simulink model "ADIA"  (R2018b)
settings: Solver=FixedStepDiscrete  StartTime=0.0  StopTime=10.0  FixedStep=0.02  RelTol=1e-3
undefined symbols (not defined in the file or in its folder): ACC_State_Active, ACC_State_BrakeOnly, ACC_State_Suspended, ACC_State_WaitingRise, ADAS_AEBBrakingProg, ADAS_DeclControlReq, ADAS_DriveOff, ADAS_ESCHoldReq_NotHold, ADASDecType_ACC, ADASDecType_AEB, ADIA_ACC_Acceleration_OOR_DecCount_C, ADIA_ACC_Acceleration_OOR_Duration_C, ADIA_ACC_Acceleration_OOR_IncCount_C, ADIA_ACC_Acceleration_OOR_LLim_C, ADIA_ACC_Acceleration_OOR_ULim_C, ADIA_ACC_AccelTrqReq_MixedDia_ULim_C, ADIA_ACC_AccelTrqReq_ULim_C, ADIA_ACC_Deceleration_Mixed_ULim_C, ADIA_ACC_Deceleration_OOR_DecCount_C, ADIA_ACC_Deceleration_OOR_Duration_C, ADIA_ACC_Deceleration_OOR_IncCount_C, ADIA_ACC_Deceleration_OOR_LLim_C, ADIA_ACC_Deceleration_OOR_ULim_C, ADIA_ACC_DriveOff_Distance_C, ADIA_ACC_DriveOff_TimeLim_C, ADIA_ACC_ReqMixed_DecCount_C, ADIA_ACC_ReqMixed_Duration_C, ADIA_ACC_ReqMixed_IncCount_C, ADIA_AccPedalRaw_MaxLim_C, ADIA_AccPedalRaw_MinLim_C, ADIA_ADAS_HoldDecReq_Set_C, ADIA_ADAS_HoldRConfirm_TimeLim_C, ADIA_ADAS_HoldVehSpd_Lim_C, ADIA_AEB_VehSpdDec_LLim_C, ADIA_AEB_VehSpdDec_ULim_C, ADIA_ASWFault_OvrdEn_C, ADIA_ASWFault_OvrdValue_C, ADIA_BatteryOutOfRange_DecCount_C, ADIA_BatteryOutOfRange_Duration_C, ADIA_BatteryOutOfRange_IncCount_C, ADIA_BattVolt_MaxLim_C, ADIA_BattVolt_MinLim_C, ADIA_BCM3_33C_InvBrkLight_DecCount_C, ADIA_BCM3_33C_InvBrkLight_Duration_C, ADIA_BCM3_33C_InvBrkLight_IncCount_C, ADIA_BCM_BattVolt_OvrdEn_C, ADIA_BCM_BattVolt_OvrdVal_C, ADIA_BCM_BrakeLampStaus_OvrdEn_C, ADIA_BCM_BrakeLampStaus_OvrdVal_C, ADIA_BCM_CHMSLStaus_OvrdEn_C, ADIA_BCM_CHMSLStaus_OvrdVal_C, ADIA_BCM_LeftTurnSwSt_OvrdEn_C, ADIA_BCM_LeftTurnSwSt_OvrdVal_C, ADIA_BCM_RightTurnSwSt_OvrdEn_C, ADIA_BCM_RightTurnSwSt_OvrdVal_C, ADIA_BCM_TurnSwFailure_DecCount_C, ADIA_BCM_TurnSwFailure_Duration_C, ADIA_BCM_TurnSwFailure_IncCount_C, ADIA_BSWFault_Ignore_C, ADIA_BSWFault_OvrdEn_C ... (+281)
libraries: simulink x208
(part 6 of 10)

== system ADIA/ADAS_Diagnostics/Diagnostics_Processing/Rationality_Diagnostics/ESC6_123_InvVehDriDirec ==
  Compare To Constant27 : simulink/Logic and Bit Operations/Compare To Constant  relop===  const=3  OutDataTypeStr=boolean
  Constant18 : Constant  Value=Constant_0
  Constant19 : Constant  Value=ADIA_ESC6_123_InvVehDriDirec_DecCount_C
  Constant20 : Constant  Value=ADIA_ESC6_123_InvVehDriDirec_IncCount_C
  Constant21 : Constant  Value=ADIA_ESC6_123_InvVehDriDirec_Duration_C
  Constant22 : Constant  Value=SYS_False
  Counter&Latch : Subsystem
  Data Store Read67 : DataStoreRead  DataStoreName=ADIAve_y_ESC_VehDrivingDirection
  Logical Operator20 : Logic  Operator=NOT  AllPortsSameDT=off  OutDataTypeStr=boolean
  ADIA_DTC_ESC6_123_InvVehDriDirec : Outport
  wires:
  Compare To Constant27/1 -> Logical Operator20/1, Counter&Latch/1(incrcondition)  "Event_OutRangePowStrSta_SetEventStatus19"
  Data Store Read67/1 -> Compare To Constant27/1  "ob_ADIAve_y_ESC_VehDrivingDirection"
  Logical Operator20/1 -> Counter&Latch/3(decrcondition)
  Constant19/1 -> Counter&Latch/4(decvalue)
  Constant20/1 -> Counter&Latch/2(incrvalue)
  Constant18/1 -> Counter&Latch/7(LatchResetCounterVal)
  Constant21/1 -> Counter&Latch/5(maxlimit)
  Constant22/1 -> Counter&Latch/6(reset)
  Counter&Latch/1(Out1) -> ADIA_DTC_ESC6_123_InvVehDriDirec/1

== system ADIA/ADAS_Diagnostics/Diagnostics_Processing/Rationality_Diagnostics/ESC6_123_InvVehHoldStas ==
  Compare To Constant45 : simulink/Logic and Bit Operations/Compare To Constant  relop===  const=3  OutDataTypeStr=boolean
  Constant18 : Constant  Value=Constant_0
  Constant19 : Constant  Value=ADIA_ESC6_123_InvVehHoldStas_DecCount_C
  Constant20 : Constant  Value=ADIA_ESC6_123_InvVehHoldStas_IncCount_C
  Constant21 : Constant  Value=ADIA_ESC6_123_InvVehHoldStas_Duration_C
  Constant22 : Constant  Value=SYS_False
  Counter&Latch : Subsystem
  Data Store Read33 : DataStoreRead  DataStoreName=ADIAve_y_ESC_VehHoldState
  Logical Operator20 : Logic  Operator=NOT  AllPortsSameDT=off  OutDataTypeStr=boolean
  ADIA_DTC_ESC6_123_InvVehHoldStas : Outport
  wires:
  Compare To Constant45/1 -> Counter&Latch/1(incrcondition), Logical Operator20/1  "Event_OutRangeHoldSta_SetEventStatus22"
  Data Store Read33/1 -> Compare To Constant45/1
  Logical Operator20/1 -> Counter&Latch/3(decrcondition)
  Constant19/1 -> Counter&Latch/4(decvalue)
  Constant20/1 -> Counter&Latch/2(incrvalue)
  Constant18/1 -> Counter&Latch/7(LatchResetCounterVal)
  Constant21/1 -> Counter&Latch/5(maxlimit)
  Constant22/1 -> Counter&Latch/6(reset)
  Counter&Latch/1(Out1) -> ADIA_DTC_ESC6_123_InvVehHoldStas/1

== system ADIA/ADAS_Diagnostics/Diagnostics_Processing/Rationality_Diagnostics/Event_Fault_ABSorESC ==
  Compare To Constant8 : simulink/Logic and Bit Operations/Compare To Constant  relop===  const=1  OutDataTypeStr=boolean
  Compare To Constant9 : simulink/Logic and Bit Operations/Compare To Constant  relop===  const=1  OutDataTypeStr=boolean
  Data Store Read52 : DataStoreRead  DataStoreName=ADIAve_y_ESC_ABSValidity
  Data Store Read53 : DataStoreRead  DataStoreName=ADIAve_y_ESC_ESCValidity
  Logical Operator20 : Logic  Operator=OR  AllPortsSameDT=off  OutDataTypeStr=boolean
  "Event_Fault_ABSorESC " : Outport
  wires:
  Data Store Read52/1 -> Compare To Constant8/1
  Compare To Constant9/1 -> Logical Operator20/2  "Event_FaulESCLamp6"
  Data Store Read53/1 -> Compare To Constant9/1
  Logical Operator20/1 -> "Event_Fault_ABSorESC "/1
  Compare To Constant8/1 -> Logical Operator20/1  "Event_FaulABSLamp5"

== system ADIA/ADAS_Diagnostics/Diagnostics_Processing/Rationality_Diagnostics/FRadar_FaultState ==
  Constant18 : Constant  Value=Constant_0
  Constant19 : Constant  Value=ADIA_FRadar_FaultState_DecCount_C
  Constant20 : Constant  Value=ADIA_FRadar_FaultState_IncCount_C
  Constant21 : Constant  Value=ADIA_FRadar_FaultState_Duration_C
  Constant22 : Constant  Value=SYS_False
  Constant37 : Constant  Value=FRadar_State_Sensoring
  Counter&Latch : Subsystem
  Data Store Read74 : DataStoreRead  DataStoreName=ADIAve_y_Radar_State
  Logical Operator20 : Logic  Operator=NOT  AllPortsSameDT=off  OutDataTypeStr=boolean
  Relational Operator37 : RelationalOperator  Operator=~=  OutDataTypeStr=boolean  RndMeth=Simplest
  ADIA_Inner_FRadar_FaultState : Outport
  wires:
  Constant37/1 -> Relational Operator37/2
  Data Store Read74/1 -> Relational Operator37/1  "ob_ADIAve_y_Radar_State"
  Logical Operator20/1 -> Counter&Latch/3(decrcondition)
  Relational Operator37/1 -> Logical Operator20/1, Counter&Latch/1(incrcondition)
  Constant19/1 -> Counter&Latch/4(decvalue)
  Constant20/1 -> Counter&Latch/2(incrvalue)
  Constant18/1 -> Counter&Latch/7(LatchResetCounterVal)
  Constant21/1 -> Counter&Latch/5(maxlimit)
  Constant22/1 -> Counter&Latch/6(reset)
  Counter&Latch/1(Out1) -> ADIA_Inner_FRadar_FaultState/1

== system ADIA/ADAS_Diagnostics/Diagnostics_Processing/Rationality_Diagnostics/MP5_366_OorAEBButton ==
  Compare To Constant50 : simulink/Logic and Bit Operations/Compare To Constant  relop===  const=3  OutDataTypeStr=boolean
  Constant18 : Constant  Value=Constant_0
  Constant19 : Constant  Value=ADIA_MP5_366_OorAEBButton_DecCount_C
  Constant20 : Constant  Value=ADIA_MP5_366_OorAEBButton_IncCount_C
  Constant21 : Constant  Value=ADIA_MP5_366_OorAEBButton_Duration_C
  Constant22 : Constant  Value=SYS_False
  Counter&Latch : Subsystem
  Data Store Read38 : DataStoreRead  DataStoreName=ADIAve_y_MP5_AEBSwitch
  Logical Operator20 : Logic  Operator=NOT  AllPortsSameDT=off  OutDataTypeStr=boolean
  ADIA_DTC_MP5_366_OorAEBButton : Outport
  wires:
  Data Store Read38/1 -> Compare To Constant50/1
  Logical Operator20/1 -> Counter&Latch/3(decrcondition)
  Compare To Constant50/1 -> Logical Operator20/1, Counter&Latch/1(incrcondition)
  Constant19/1 -> Counter&Latch/4(decvalue)
  Constant20/1 -> Counter&Latch/2(incrvalue)
  Constant18/1 -> Counter&Latch/7(LatchResetCounterVal)
  Constant21/1 -> Counter&Latch/5(maxlimit)
  Constant22/1 -> Counter&Latch/6(reset)
  Counter&Latch/1(Out1) -> ADIA_DTC_MP5_366_OorAEBButton/1

== system ADIA/ADAS_Diagnostics/Diagnostics_Processing/Rationality_Diagnostics/MP5_366_OorFCWButton ==
  Compare To Constant51 : simulink/Logic and Bit Operations/Compare To Constant  relop===  const=3  OutDataTypeStr=boolean
  Constant18 : Constant  Value=Constant_0
  Constant19 : Constant  Value=ADIA_MP5_366_OorFCWButton_DecCount_C
  Constant20 : Constant  Value=ADIA_MP5_366_OorFCWButton_IncCount_C
  Constant21 : Constant  Value=ADIA_MP5_366_OorFCWButton_Duration_C
  Constant22 : Constant  Value=SYS_False
  Counter&Latch : Subsystem
  Data Store Read37 : DataStoreRead  DataStoreName=ADIAve_y_MP5_FCWSwitch
  Logical Operator20 : Logic  Operator=NOT  AllPortsSameDT=off  OutDataTypeStr=boolean
  ADIA_DTC_MP5_366_OorFCWButton : Outport
  wires:
  Data Store Read37/1 -> Compare To Constant51/1
  Logical Operator20/1 -> Counter&Latch/3(decrcondition)
  Compare To Constant51/1 -> Counter&Latch/1(incrcondition), Logical Operator20/1
  Constant19/1 -> Counter&Latch/4(decvalue)
  Constant20/1 -> Counter&Latch/2(incrvalue)
  Constant18/1 -> Counter&Latch/7(LatchResetCounterVal)
  Constant21/1 -> Counter&Latch/5(maxlimit)
  Constant22/1 -> Counter&Latch/6(reset)
  Counter&Latch/1(Out1) -> ADIA_DTC_MP5_366_OorFCWButton/1

== system ADIA/ADAS_Diagnostics/Diagnostics_Processing/Rationality_Diagnostics/MP5_413_OorISAMode ==
  Compare To Constant31 : simulink/Logic and Bit Operations/Compare To Constant  relop===  const=3  OutDataTypeStr=boolean
  Constant18 : Constant  Value=Constant_0
  Constant19 : Constant  Value=ADIA_MP5_413_OorISAMode_DecCount_C
  Constant20 : Constant  Value=ADIA_MP5_413_OorISAMode_IncCount_C
  Constant21 : Constant  Value=ADIA_MP5_413_OorISAMode_Duration_C
  Constant22 : Constant  Value=SYS_False
  Counter&Latch : Subsystem
  Data Store Read71 : DataStoreRead  DataStoreName=ADIAve_y_Mp5_ISAMode
  Logical Operator20 : Logic  Operator=NOT  AllPortsSameDT=off  OutDataTypeStr=boolean
  ADIA_DTC_GW_MP5_413_OorISAMode : Outport
  wires:
  Compare To Constant31/1 -> Logical Operator20/1, Counter&Latch/1(incrcondition)  "Event_OutRangePowStrSta_SetEventStatus19"
  Data Store Read71/1 -> Compare To Constant31/1  "ob_ADIAve_y_Mp5_ISAMode"
  Logical Operator20/1 -> Counter&Latch/3(decrcondition)
  Constant19/1 -> Counter&Latch/4(decvalue)
  Constant20/1 -> Counter&Latch/2(incrvalue)
  Constant18/1 -> Counter&Latch/7(LatchResetCounterVal)
  Constant21/1 -> Counter&Latch/5(maxlimit)
  Constant22/1 -> Counter&Latch/6(reset)
  Counter&Latch/1(Out1) -> ADIA_DTC_GW_MP5_413_OorISAMode/1

== system ADIA/ADAS_Diagnostics/Diagnostics_Processing/Rationality_Diagnostics/MP5_413_OorLKAMode ==
  Compare To Constant49 : simulink/Logic and Bit Operations/Compare To Constant  relop=>=  const=6  OutDataTypeStr=boolean
  Constant18 : Constant  Value=Constant_0
  Constant19 : Constant  Value=ADIA_MP5_413_OorLKAMode_DecCount_C
  Constant20 : Constant  Value=ADIA_MP5_413_OorLKAMode_IncCount_C
  Constant21 : Constant  Value=ADIA_MP5_413_OorLKAMode_Duration_C
  Constant22 : Constant  Value=SYS_False
  Counter&Latch : Subsystem
  Data Store Read39 : DataStoreRead  DataStoreName=ADIAve_y_Mp5_LSSMode
  Logical Operator20 : Logic  Operator=NOT  AllPortsSameDT=off  OutDataTypeStr=boolean
  ADIA_DTC_GW_MP5_413_OorLKAMode : Outport
  wires:
  Data Store Read39/1 -> Compare To Constant49/1
  Logical Operator20/1 -> Counter&Latch/3(decrcondition)
  Compare To Constant49/1 -> Counter&Latch/1(incrcondition), Logical Operator20/1
  Constant19/1 -> Counter&Latch/4(decvalue)
  Constant20/1 -> Counter&Latch/2(incrvalue)
  Constant18/1 -> Counter&Latch/7(LatchResetCounterVal)
  Constant21/1 -> Counter&Latch/5(maxlimit)
  Constant22/1 -> Counter&Latch/6(reset)
  Counter&Latch/1(Out1) -> ADIA_DTC_GW_MP5_413_OorLKAMode/1

== system ADIA/ADAS_Diagnostics/Diagnostics_Processing/Rationality_Diagnostics/SAS_A5_InvOorSteAngle ==
  Abs6 : Abs
  Constant15 : Constant  Value=ADIA_SAS_SteerAngle_MaxLim_C
  Constant18 : Constant  Value=Constant_0
  Constant19 : Constant  Value=ADIA_SAS_A5_InvOorSteAngle_DecCount_C
  Constant20 : Constant  Value=ADIA_SAS_A5_InvOorSteAngle_IncCount_C
  Constant21 : Constant  Value=ADIA_SAS_A5_InvOorSteAngle_Duration_C
  Constant22 : Constant  Value=SYS_False
  Counter&Latch : Subsystem
  Data Store Read28 : DataStoreRead  DataStoreName=ADIAve_g_SAS_SteerAngle
  Logical Operator20 : Logic  Operator=NOT  AllPortsSameDT=off  OutDataTypeStr=boolean
  Relational Operator13 : RelationalOperator  Operator=>  OutDataTypeStr=boolean  RndMeth=Simplest
  ADIA_DTC_SAS_A5_InvOorSteAngle : Outport
  wires:
  Data Store Read28/1 -> Abs6/1
  Abs6/1 -> Relational Operator13/1
  Constant15/1 -> Relational Operator13/2
  Logical Operator20/1 -> Counter&Latch/3(decrcondition)
  Relational Operator13/1 -> Logical Operator20/1, Counter&Latch/1(incrcondition)
  Constant19/1 -> Counter&Latch/4(decvalue)
  Constant20/1 -> Counter&Latch/2(incrvalue)
  Constant18/1 -> Counter&Latch/7(LatchResetCounterVal)
  Constant21/1 -> Counter&Latch/5(maxlimit)
  Constant22/1 -> Counter&Latch/6(reset)
  Counter&Latch/1(Out1) -> ADIA_DTC_SAS_A5_InvOorSteAngle/1

== system ADIA/ADAS_Diagnostics/Diagnostics_Processing/Rationality_Diagnostics/SAS_A5_InvRotSpeed ==
  Abs7 : Abs
  Constant16 : Constant  Value=ADIA_SAS_SteerRotSpd_MaxLim_C
  Constant18 : Constant  Value=Constant_0
  Constant19 : Constant  Value=ADIA_SAS_A5_InvRotSpeed_DecCount_C
  Constant20 : Constant  Value=ADIA_SAS_A5_InvRotSpeed_IncCount_C
  Constant21 : Constant  Value=ADIA_SAS_A5_InvRotSpeed_Duration_C
  Constant22 : Constant  Value=SYS_False
  Counter&Latch : Subsystem
  Data Store Read27 : DataStoreRead  DataStoreName=ADIAve_g_SAS_SteerRotSpd
  Logical Operator20 : Logic  Operator=NOT  AllPortsSameDT=off  OutDataTypeStr=boolean
  Relational Operator14 : RelationalOperator  Operator=>  OutDataTypeStr=boolean  RndMeth=Simplest
  ADIA_DTC_SASInfo_A5_InvRotSpeed : Outport
  wires:
  Data Store Read27/1 -> Abs7/1
  Constant16/1 -> Relational Operator14/2
  Abs7/1 -> Relational Operator14/1
  Logical Operator20/1 -> Counter&Latch/3(decrcondition)
  Relational Operator14/1 -> Counter&Latch/1(incrcondition), Logical Operator20/1
  Constant19/1 -> Counter&Latch/4(decvalue)
  Constant20/1 -> Counter&Latch/2(incrvalue)
  Constant18/1 -> Counter&Latch/7(LatchResetCounterVal)
  Constant21/1 -> Counter&Latch/5(maxlimit)
  Constant22/1 -> Counter&Latch/6(reset)
  Counter&Latch/1(Out1) -> ADIA_DTC_SASInfo_A5_InvRotSpeed/1

== system ADIA/ADAS_Diagnostics/Diagnostics_Processing/Rationality_Diagnostics/SCC_309_OorACCButton ==
  Constant18 : Constant  Value=Constant_0
  Constant19 : Constant  Value=ADIA_SCC_309_OorACCButton_DecCount_C
  Constant20 : Constant  Value=ADIA_SCC_309_OorACCButton_IncCount_C
  Constant21 : Constant  Value=ADIA_SCC_309_OorACCButton_Duration_C
  Constant22 : Constant  Value=SYS_False
  Constant42 : Constant  Value=IVI_LeftSteeringWhlSw_Fault
  Counter&Latch : Subsystem
  Data Store Read36 : DataStoreRead  DataStoreName=ADIAve_y_SCC_LeftSteerWhlSw
  Logical Operator20 : Logic  Operator=NOT  AllPortsSameDT=off  OutDataTypeStr=boolean
  Relational Operator42 : RelationalOperator  Operator===  OutDataTypeStr=boolean  RndMeth=Simplest
  ADIA_DTC_SCC_309_OorACCButton : Outport
  wires:
  Data Store Read36/1 -> Relational Operator42/1
  Constant42/1 -> Relational Operator42/2
  Logical Operator20/1 -> Counter&Latch/3(decrcondition)
  Relational Operator42/1 -> Logical Operator20/1, Counter&Latch/1(incrcondition)
  Constant19/1 -> Counter&Latch/4(decvalue)
  Constant20/1 -> Counter&Latch/2(incrvalue)
  Constant18/1 -> Counter&Latch/7(LatchResetCounterVal)
  Constant21/1 -> Counter&Latch/5(maxlimit)
  Constant22/1 -> Counter&Latch/6(reset)
  Counter&Latch/1(Out1) -> ADIA_DTC_SCC_309_OorACCButton/1

== system ADIA/ADAS_Diagnostics/Diagnostics_Processing/Rationality_Diagnostics/Subsystem1 ==
  Constant18 : Constant  Value=Constant_0
  Constant19 : Constant  Value=ADIA_ESC_EPBErrorStatus_DecCount_C
  Constant20 : Constant  Value=ADIA_ESC_EPBErrorStatus_IncCount_C
  Constant21 : Constant  Value=ADIA_ESC_EPBErrorStatus_Duration_C
  Constant22 : Constant  Value=SYS_False
  Counter&Latch : Subsystem
  Data Store Read69 : DataStoreRead  DataStoreName=ADIAve_y_ESC_EPBErrorState
  ESC_EPBError : Constant  Value=ESC_EPBError
  Logical Operator20 : Logic  Operator=NOT  AllPortsSameDT=off  OutDataTypeStr=boolean
  Relational Operator16 : RelationalOperator  Operator===  OutDataTypeStr=boolean  RndMeth=Simplest
  ADIA_DTC_ESC_EPBErrorStatus : Outport
  wires:
  Data Store Read69/1 -> Relational Operator16/1
  ESC_EPBError/1 -> Relational Operator16/2
  Logical Operator20/1 -> Counter&Latch/3(decrcondition)
  Relational Operator16/1 -> Logical Operator20/1, Counter&Latch/1(incrcondition)
  Constant19/1 -> Counter&Latch/4(decvalue)
  Constant20/1 -> Counter&Latch/2(incrvalue)
  Constant18/1 -> Counter&Latch/7(LatchResetCounterVal)
  Constant21/1 -> Counter&Latch/5(maxlimit)
  Constant22/1 -> Counter&Latch/6(reset)
  Counter&Latch/1(Out1) -> ADIA_DTC_ESC_EPBErrorStatus/1

== system ADIA/ADAS_Diagnostics/Diagnostics_Processing/Rationality_Diagnostics/Subsystem2 ==
  note: SAS_SASFailureSts = 0 表示fault
  Compare To Constant28 : simulink/Logic and Bit Operations/Compare To Constant  relop===  const=0  OutDataTypeStr=boolean
  Constant18 : Constant  Value=Constant_0
  Constant19 : Constant  Value=ADIA_SAS_SASFailureSts_DecCount_C
  Constant20 : Constant  Value=ADIA_SAS_SASFailureSts_IncCount_C
  Constant21 : Constant  Value=ADIA_SAS_SASFailureSts_Duration_C
  Constant22 : Constant  Value=SYS_False
  Counter&Latch : Subsystem
  Data Store Read76 : DataStoreRead  DataStoreName=ADIAve_y_SAS_SASFailureSt
  Logical Operator20 : Logic  Operator=NOT  AllPortsSameDT=off  OutDataTypeStr=boolean
  ADIA_DTC_SAS_SASFailureSts : Outport
  wires:
  Data Store Read76/1 -> Compare To Constant28/1
  Logical Operator20/1 -> Counter&Latch/3(decrcondition)
  Compare To Constant28/1 -> Logical Operator20/1, Counter&Latch/1(incrcondition)
  Constant19/1 -> Counter&Latch/4(decvalue)
  Constant20/1 -> Counter&Latch/2(incrvalue)
  Constant18/1 -> Counter&Latch/7(LatchResetCounterVal)
  Constant21/1 -> Counter&Latch/5(maxlimit)
  Constant22/1 -> Counter&Latch/6(reset)
  Counter&Latch/1(Out1) -> ADIA_DTC_SAS_SASFailureSts/1

== system ADIA/ADAS_Diagnostics/Diagnostics_Processing/Rationality_Diagnostics/Subsystem3 ==
  Constant1 : Constant  Value=BCM_TurnSwitch_Fault
  Constant18 : Constant  Value=Constant_0
  Constant19 : Constant  Value=ADIA_BCM_TurnSwFailure_DecCount_C
  Constant20 : Constant  Value=ADIA_BCM_TurnSwFailure_IncCount_C
  Constant21 : Constant  Value=ADIA_BCM_TurnSwFailure_Duration_C
  Constant22 : Constant  Value=SYS_False
  Constant23 : Constant  Value=BCM_TurnSwitch_Invalid
  Counter&Latch : Subsystem
  Data Store Read77 : DataStoreRead  DataStoreName=ADIAve_y_BCM_LeftTurnSwSt
  Data Store Read78 : DataStoreRead  DataStoreName=ADIAve_y_BCM_RightTurnSwSt
  Logical Operator20 : Logic  Operator=NOT  AllPortsSameDT=off  OutDataTypeStr=boolean
  Logical Operator4 : Logic  Operator=OR  AllPortsSameDT=off  OutDataTypeStr=boolean
  Logical Operator6 : Logic  Operator=OR  AllPortsSameDT=off  OutDataTypeStr=boolean
  Logical Operator7 : Logic  Operator=OR  AllPortsSameDT=off  OutDataTypeStr=boolean
  Relational Operator{17..20} (4 alike) : RelationalOperator  Operator===  OutDataTypeStr=boolean  RndMeth=Simplest
  ADIA_DTC_BCM_TurnSwFailure : Outport
  wires:
  Relational Operator19/1 -> Logical Operator6/1
  Relational Operator18/1 -> Logical Operator4/2
  Relational Operator17/1 -> Logical Operator4/1
  Logical Operator6/1 -> Logical Operator7/2
  Constant1/1 -> Relational Operator19/2, Relational Operator17/2
  Constant23/1 -> Relational Operator20/2, Relational Operator18/2
  Data Store Read77/1 -> Relational Operator18/1, Relational Operator17/1
  Data Store Read78/1 -> Relational Operator20/1, Relational Operator19/1
  Logical Operator4/1 -> Logical Operator7/1
  Relational Operator20/1 -> Logical Operator6/2
  Logical Operator20/1 -> Counter&Latch/3(decrcondition)
  Logical Operator7/1 -> Logical Operator20/1, Counter&Latch/1(incrcondition)
  Constant19/1 -> Counter&Latch/4(decvalue)
  Constant20/1 -> Counter&Latch/2(incrvalue)
  Constant18/1 -> Counter&Latch/7(LatchResetCounterVal)
  Constant21/1 -> Counter&Latch/5(maxlimit)
  Constant22/1 -> Counter&Latch/6(reset)
  Counter&Latch/1(Out1) -> ADIA_DTC_BCM_TurnSwFailure/1

== system ADIA/ADAS_Diagnostics/Diagnostics_Processing/Rationality_Diagnostics/TCU1_93_InvOorGear ==
  Constant18 : Constant  Value=Constant_0
  Constant19 : Constant  Value=ADIA_TCU1_93_InvOorGear_DecCount_C
  Constant20 : Constant  Value=ADIA_TCU1_93_InvOorGear_IncCount_C
  Constant21 : Constant  Value=ADIA_TCU1_93_InvOorGear_Duration_C
  Constant22 : Constant  Value=SYS_False
  Constant41 : Constant  Value=TCU_ActualGear_Invalid
  Counter&Latch : Subsystem
  Data Store Read35 : DataStoreRead  DataStoreName=ADIAve_y_TCU_ActualGear
  Logical Operator20 : Logic  Operator=NOT  AllPortsSameDT=off  OutDataTypeStr=boolean
  Relational Operator41 : RelationalOperator  Operator===  OutDataTypeStr=boolean  RndMeth=Simplest
  ADIA_DTC_TCU1_93_InvOorGear : Outport
  wires:
  Constant41/1 -> Relational Operator41/2
  Data Store Read35/1 -> Relational Operator41/1
  Logical Operator20/1 -> Counter&Latch/3(decrcondition)
  Relational Operator41/1 -> Logical Operator20/1, Counter&Latch/1(incrcondition)
  Constant19/1 -> Counter&Latch/4(decvalue)
  Constant20/1 -> Counter&Latch/2(incrvalue)
  Constant18/1 -> Counter&Latch/7(LatchResetCounterVal)
  Constant21/1 -> Counter&Latch/5(maxlimit)
  Constant22/1 -> Counter&Latch/6(reset)
  Counter&Latch/1(Out1) -> ADIA_DTC_TCU1_93_InvOorGear/1

== system ADIA/ADAS_Diagnostics/Diagnostics_Processing/Subsystem1/16Bits_Set1 ==
  Bit1 : Inport  OutDataTypeStr=boolean
  Bit2 : Inport  Port=2  OutDataTypeStr=boolean
  Bit3 : Inport  Port=3  OutDataTypeStr=boolean
  Bit4 : Inport  Port=4  OutDataTypeStr=boolean
  Bit5 : Inport  Port=5  OutDataTypeStr=boolean
  Bit6 : Inport  Port=6  OutDataTypeStr=boolean
  Bit7 : Inport  Port=7  OutDataTypeStr=boolean
  Bit8 : Inport  Port=8  OutDataTypeStr=boolean
  Bit9 : Inport  Port=9  OutDataTypeStr=boolean
  Bit10 : Inport  Port=10  OutDataTypeStr=boolean
  Bit11 : Inport  Port=11  OutDataTypeStr=boolean
  Bit12 : Inport  Port=12  OutDataTypeStr=boolean
  Bit13 : Inport  Port=13  OutDataTypeStr=boolean
  Bit14 : Inport  Port=14  OutDataTypeStr=boolean
  Bit15 : Inport  Port=15  OutDataTypeStr=boolean
  Bit16 : Inport  Port=16  OutDataTypeStr=boolean
  8Bits_Set : Subsystem
  8Bits_Set1 : Subsystem
  Add : Sum
  Data Type Conversion : DataTypeConversion  OutDataTypeStr=uint16
  Data Type Conversion1 : DataTypeConversion  OutDataTypeStr=uint16
  Shift Arithmetic : ArithShift  BitShiftNumber=8  BitShiftDirection=Left
  Index_16Bits : Outport  OutDataTypeStr=uint16
  wires:
  Data Type Conversion1/1 -> Shift Arithmetic/1
  Data Type Conversion/1 -> Add/1
  Bit16/1 -> 8Bits_Set1/8(Bit8)
  Bit15/1 -> 8Bits_Set1/7(Bit7)
  Bit14/1 -> 8Bits_Set1/6(Bit6)
  Bit13/1 -> 8Bits_Set1/5(Bit5)
  Bit12/1 -> 8Bits_Set1/4(Bit4)
  Bit11/1 -> 8Bits_Set1/3(Bit3)
  Bit10/1 -> 8Bits_Set1/2(Bit2)
  Bit9/1 -> 8Bits_Set1/1(Bit1)
  Add/1 -> Index_16Bits/1
  8Bits_Set/1(Index_8Bits) -> Data Type Conversion/1
  Shift Arithmetic/1 -> Add/2
  8Bits_Set1/1(Index_8Bits) -> Data Type Conversion1/1
  Bit8/1 -> 8Bits_Set/8(Bit8)
  Bit7/1 -> 8Bits_Set/7(Bit7)
  Bit6/1 -> 8Bits_Set/6(Bit6)
  Bit5/1 -> 8Bits_Set/5(Bit5)
  Bit4/1 -> 8Bits_Set/4(Bit4)
  Bit3/1 -> 8Bits_Set/3(Bit3)
  Bit2/1 -> 8Bits_Set/2(Bit2)
  Bit1/1 -> 8Bits_Set/1(Bit1)

== system ADIA/ADAS_Diagnostics/Diagnostics_Processing/Subsystem1/16Bits_Set2 ==
  Bit0 : Inport  OutDataTypeStr=boolean
  Bit1 : Inport  Port=2  OutDataTypeStr=boolean
  Bit2 : Inport  Port=3  OutDataTypeStr=boolean
  Bit3 : Inport  Port=4  OutDataTypeStr=boolean
  Bit4 : Inport  Port=5  OutDataTypeStr=boolean
  Bit5 : Inport  Port=6  OutDataTypeStr=boolean
  Bit6 : Inport  Port=7  OutDataTypeStr=boolean
  Bit7 : Inport  Port=8  OutDataTypeStr=boolean
  Bit8 : Inport  Port=9  OutDataTypeStr=boolean
  Bit9 : Inport  Port=10  OutDataTypeStr=boolean
  Bit10 : Inport  Port=11  OutDataTypeStr=boolean
  Bit11 : Inport  Port=12  OutDataTypeStr=boolean
  Bit12 : Inport  Port=13  OutDataTypeStr=boolean
  Bit13 : Inport  Port=14  OutDataTypeStr=boolean
  Bit14 : Inport  Port=15  OutDataTypeStr=boolean
  Bit15 : Inport  Port=16  OutDataTypeStr=boolean
  8Bits_Set : Subsystem
  8Bits_Set1 : Subsystem
  Add : Sum
  Data Type Conversion : DataTypeConversion  OutDataTypeStr=uint16
  Data Type Conversion1 : DataTypeConversion  OutDataTypeStr=uint16
  Shift Arithmetic : ArithShift  BitShiftNumber=8  BitShiftDirection=Left
  Index_16Bits : Outport  OutDataTypeStr=uint16
  wires:
  8Bits_Set1/1(Index_8Bits) -> Data Type Conversion1/1
  Shift Arithmetic/1 -> Add/2
  8Bits_Set/1(Index_8Bits) -> Data Type Conversion/1
  Add/1 -> Index_16Bits/1
  Data Type Conversion/1 -> Add/1
  Data Type Conversion1/1 -> Shift Arithmetic/1
  Bit0/1 -> 8Bits_Set/1(Bit0)
  Bit1/1 -> 8Bits_Set/2(Bit1)
  Bit2/1 -> 8Bits_Set/3(Bit2)
  Bit3/1 -> 8Bits_Set/4(Bit3)
  Bit4/1 -> 8Bits_Set/5(Bit4)
  Bit5/1 -> 8Bits_Set/6(Bit5)
  Bit6/1 -> 8Bits_Set/7(Bit6)
  Bit7/1 -> 8Bits_Set/8(Bit7)
  Bit8/1 -> 8Bits_Set1/1(Bit0)
  Bit9/1 -> 8Bits_Set1/2(Bit1)
  Bit10/1 -> 8Bits_Set1/3(Bit2)
  Bit11/1 -> 8Bits_Set1/4(Bit3)
  Bit12/1 -> 8Bits_Set1/5(Bit4)
  Bit13/1 -> 8Bits_Set1/6(Bit5)
  Bit14/1 -> 8Bits_Set1/7(Bit6)
  Bit15/1 -> 8Bits_Set1/8(Bit7)

== system ADIA/ADAS_Diagnostics/Diagnostics_Processing/Subsystem3/16Bits_Set ==
  Bit0 : Inport  OutDataTypeStr=boolean
  Bit1 : Inport  Port=2  OutDataTypeStr=boolean
  Bit2 : Inport  Port=3  OutDataTypeStr=boolean
  Bit3 : Inport  Port=4  OutDataTypeStr=boolean
  Bit4 : Inport  Port=5  OutDataTypeStr=boolean
  Bit5 : Inport  Port=6  OutDataTypeStr=boolean
  Bit6 : Inport  Port=7  OutDataTypeStr=boolean
  Bit7 : Inport  Port=8  OutDataTypeStr=boolean
  Bit8 : Inport  Port=9  OutDataTypeStr=boolean
  Bit9 : Inport  Port=10  OutDataTypeStr=boolean
  Bit10 : Inport  Port=11  OutDataTypeStr=boolean
  Bit11 : Inport  Port=12  OutDataTypeStr=boolean
  Bit12 : Inport  Port=13  OutDataTypeStr=boolean
  Bit13 : Inport  Port=14  OutDataTypeStr=boolean
  Bit14 : Inport  Port=15  OutDataTypeStr=boolean
  Bit15 : Inport  Port=16  OutDataTypeStr=boolean
  8Bits_Set : Subsystem
  8Bits_Set1 : Subsystem
  Add : Sum
  Data Type Conversion : DataTypeConversion  OutDataTypeStr=uint16
  Data Type Conversion1 : DataTypeConversion  OutDataTypeStr=uint16
  Shift Arithmetic : ArithShift  BitShiftNumber=8  BitShiftDirection=Left
  Index_16Bits : Outport  OutDataTypeStr=uint16
  wires:
  Bit15/1 -> 8Bits_Set1/8(Bit7)
  Bit14/1 -> 8Bits_Set1/7(Bit6)
  Bit13/1 -> 8Bits_Set1/6(Bit5)
  Bit12/1 -> 8Bits_Set1/5(Bit4)
  Bit11/1 -> 8Bits_Set1/4(Bit3)
  Bit10/1 -> 8Bits_Set1/3(Bit2)
  Bit9/1 -> 8Bits_Set1/2(Bit1)
  Bit8/1 -> 8Bits_Set1/1(Bit0)
  Bit7/1 -> 8Bits_Set/8(Bit7)
  Bit6/1 -> 8Bits_Set/7(Bit6)
  Bit5/1 -> 8Bits_Set/6(Bit5)
  Bit4/1 -> 8Bits_Set/5(Bit4)
  Bit3/1 -> 8Bits_Set/4(Bit3)
  Bit2/1 -> 8Bits_Set/3(Bit2)
  Bit1/1 -> 8Bits_Set/2(Bit1)
  Bit0/1 -> 8Bits_Set/1(Bit0)
  Data Type Conversion1/1 -> Shift Arithmetic/1
  Data Type Conversion/1 -> Add/1
  Add/1 -> Index_16Bits/1
  8Bits_Set/1(Index_8Bits) -> Data Type Conversion/1
  Shift Arithmetic/1 -> Add/2
  8Bits_Set1/1(Index_8Bits) -> Data Type Conversion1/1

== system ADIA/ADAS_Diagnostics/Diagnostics_Processing/Subsystem3/16Bits_Set1 ==
  Bit1 : Inport  OutDataTypeStr=boolean
  Bit2 : Inport  Port=2  OutDataTypeStr=boolean
  Bit3 : Inport  Port=3  OutDataTypeStr=boolean
  Bit4 : Inport  Port=4  OutDataTypeStr=boolean
  Bit5 : Inport  Port=5  OutDataTypeStr=boolean
  Bit6 : Inport  Port=6  OutDataTypeStr=boolean
  Bit7 : Inport  Port=7  OutDataTypeStr=boolean
  Bit8 : Inport  Port=8  OutDataTypeStr=boolean
  Bit9 : Inport  Port=9  OutDataTypeStr=boolean
  Bit10 : Inport  Port=10  OutDataTypeStr=boolean
  Bit11 : Inport  Port=11  OutDataTypeStr=boolean
  Bit12 : Inport  Port=12  OutDataTypeStr=boolean
  Bit13 : Inport  Port=13  OutDataTypeStr=boolean
  Bit14 : Inport  Port=14  OutDataTypeStr=boolean
  Bit15 : Inport  Port=15  OutDataTypeStr=boolean
  Bit16 : Inport  Port=16  OutDataTypeStr=boolean
  8Bits_Set : Subsystem
  8Bits_Set1 : Subsystem
  Add : Sum
  Data Type Conversion : DataTypeConversion  OutDataTypeStr=uint16
  Data Type Conversion1 : DataTypeConversion  OutDataTypeStr=uint16
  Shift Arithmetic : ArithShift  BitShiftNumber=8  BitShiftDirection=Left
  Index_16Bits : Outport  OutDataTypeStr=uint16
  wires:
  Bit1/1 -> 8Bits_Set/1(Bit1)
  Bit2/1 -> 8Bits_Set/2(Bit2)
  Bit3/1 -> 8Bits_Set/3(Bit3)
  Bit4/1 -> 8Bits_Set/4(Bit4)
  Bit5/1 -> 8Bits_Set/5(Bit5)
  Bit6/1 -> 8Bits_Set/6(Bit6)
  Bit7/1 -> 8Bits_Set/7(Bit7)
  Bit8/1 -> 8Bits_Set/8(Bit8)
  8Bits_Set1/1(Index_8Bits) -> Data Type Conversion1/1
  Shift Arithmetic/1 -> Add/2
  8Bits_Set/1(Index_8Bits) -> Data Type Conversion/1
  Add/1 -> Index_16Bits/1
  Bit9/1 -> 8Bits_Set1/1(Bit1)
  Bit10/1 -> 8Bits_Set1/2(Bit2)
  Bit11/1 -> 8Bits_Set1/3(Bit3)
  Bit12/1 -> 8Bits_Set1/4(Bit4)
  Bit13/1 -> 8Bits_Set1/5(Bit5)
  Bit14/1 -> 8Bits_Set1/6(Bit6)
  Bit15/1 -> 8Bits_Set1/7(Bit7)
  Bit16/1 -> 8Bits_Set1/8(Bit8)
  Data Type Conversion/1 -> Add/1
  Data Type Conversion1/1 -> Shift Arithmetic/1

== system ADIA/ADAS_Diagnostics/Diagnostics_Processing/DTC_ACC_Mixed_Mode_Conflict/Subsystem/Latch  ==
  Input : Inport
  Latch Reset : Inport  Port=2
  Constant11 : Constant  Value=0  OutDataTypeStr=Inherit: Inherit via back propagation
  Constant12 : Constant  OutDataTypeStr=Inherit: Inherit via back propagation
  Switch : Switch  Threshold=1  OutDataTypeStr=Inherit: Inherit via back propagation  SaturateOnIntegerOverflow=on  InputSameDT=on
  Switch1 : Switch  Threshold=1  OutDataTypeStr=Inherit: Inherit via back propagation  SaturateOnIntegerOverflow=on  InputSameDT=on
  Unit Delay1 : UnitDelay  SampleTime=-1
  Output : Outport  InitialOutput=0
  wires:
  Constant12/1 -> Switch1/1
  Constant11/1 -> Switch/1
  Input/1 -> Switch1/2
  Unit Delay1/1 -> Switch1/3
  Switch/1 -> Unit Delay1/1, Output/1
  Latch Reset/1 -> Switch/2
  Switch1/1 -> Switch/3

== system ADIA/ADAS_Diagnostics/Diagnostics_Processing/DTC_ACC_Mixed_Mode_Conflict/Subsystem/Timer1 ==
  incrcondition : Inport
  incrvalue : Inport  Port=2
  decr condition : Inport  Port=3
  decvalue : Inport  Port=4
  maxlimit : Inport  Port=5
  reset : Inport  Port=6
  Constant{,1..3} (4 alike) : Constant  Value=0  OutDataTypeStr=Inherit: Inherit via back propagation
  MinMax1 : MinMax  Inputs=2  OutDataTypeStr=Inherit: Inherit via back propagation  InputSameDT=on
  MinMax2 : MinMax  Function=max  Inputs=2  OutDataTypeStr=Inherit: Inherit via back propagation  InputSameDT=on
  Relational Operator : RelationalOperator  OutDataTypeStr=boolean  RndMeth=Nearest
  Sum : Sum  Inputs=++-  OutDataTypeStr=Inherit: Inherit via back propagation  InputSameDT=on
  Unit Delay : UnitDelay  SampleTime=-1
  dec switch : Switch  Criteria=u2 ~= 0  Threshold=1  OutDataTypeStr=Inherit: Inherit via back propagation  InputSameDT=on
  inc switch : Switch  Criteria=u2 ~= 0  Threshold=1  OutDataTypeStr=Inherit: Inherit via back propagation  InputSameDT=on
  reset switch : Switch  Criteria=u2 ~= 0  Threshold=1  OutDataTypeStr=Inherit: Inherit via back propagation  InputSameDT=on
  counter out : Outport
  counter_status : Outport  Port=2
  wires:
  decvalue/1 -> dec switch/1
  Relational Operator/1 -> counter_status/1
  Constant3/1 -> reset switch/1
  inc switch/1 -> Sum/2
  Sum/1 -> MinMax2/2
  maxlimit/1 -> MinMax1/2, Relational Operator/2
  Constant2/1 -> MinMax2/1
  reset switch/1 -> counter out/1, Relational Operator/1, Unit Delay/1
  Unit Delay/1 -> Sum/1
  reset/1 -> reset switch/2
  Constant/1 -> inc switch/3
  MinMax2/1 -> MinMax1/1
  incrvalue/1 -> inc switch/1
  MinMax1/1 -> reset switch/3
  dec switch/1 -> Sum/3
  Constant1/1 -> dec switch/3
  decr condition/1 -> dec switch/2
  incrcondition/1 -> inc switch/2

== system ADIA/ADAS_Diagnostics/Diagnostics_Processing/Rationality_Diagnostics/BatteryOutOfRange/Counter&Latch ==
  incrcondition : Inport
  incrvalue : Inport  Port=2
  decrcondition : Inport  Port=3
  decvalue : Inport  Port=4
  maxlimit : Inport  Port=5
  reset : Inport  Port=6
  LatchResetCounterVal : Inport  Port=7
  "Latch " : Subsystem
  Relational Operator16 : RelationalOperator  Operator=<=  OutDataTypeStr=boolean  RndMeth=Simplest
  Timer1 : Subsystem
  Out1 : Outport
  wires:
  Timer1/2(counter_status) -> "Latch "/1(Input)
  Timer1/1(counter out) -> Relational Operator16/1
  LatchResetCounterVal/1 -> Relational Operator16/2
  incrcondition/1 -> Timer1/1(incrcondition)
  incrvalue/1 -> Timer1/2(incrvalue)
  Relational Operator16/1 -> "Latch "/2(Latch Reset)
  "Latch "/1(Output) -> Out1/1
  maxlimit/1 -> Timer1/5(maxlimit)
  decrcondition/1 -> Timer1/3(decrcondition)
  reset/1 -> Timer1/6(reset)
  decvalue/1 -> Timer1/4(decvalue)

== system ADIA/ADAS_Diagnostics/Diagnostics_Processing/Rationality_Diagnostics/CameraSystemError/Counter&Latch ==
  incrcondition : Inport
  incrvalue : Inport  Port=2
  decrcondition : Inport  Port=3
  decvalue : Inport  Port=4
  maxlimit : Inport  Port=5
  reset : Inport  Port=6
  LatchResetCounterVal : Inport  Port=7
  "Latch " : Subsystem
  Relational Operator16 : RelationalOperator  Operator=<=  OutDataTypeStr=boolean  RndMeth=Simplest
  Timer1 : Subsystem
  Out1 : Outport
  wires:
  Timer1/2(counter_status) -> "Latch "/1(Input)
  Timer1/1(counter out) -> Relational Operator16/1
  LatchResetCounterVal/1 -> Relational Operator16/2
  incrcondition/1 -> Timer1/1(incrcondition)
  incrvalue/1 -> Timer1/2(incrvalue)
  Relational Operator16/1 -> "Latch "/2(Latch Reset)
  "Latch "/1(Output) -> Out1/1
  maxlimit/1 -> Timer1/5(maxlimit)
  decrcondition/1 -> Timer1/3(decrcondition)
  reset/1 -> Timer1/6(reset)
  decvalue/1 -> Timer1/4(decvalue)

== system ADIA/ADAS_Diagnostics/Diagnostics_Processing/Rationality_Diagnostics/DTC_BCM3_33C_InvBrkLight/Counter&Latch ==
  incrcondition : Inport
  incrvalue : Inport  Port=2
  decrcondition : Inport  Port=3
  decvalue : Inport  Port=4
  maxlimit : Inport  Port=5
  reset : Inport  Port=6
  LatchResetCounterVal : Inport  Port=7
  "Latch " : Subsystem
  Relational Operator16 : RelationalOperator  Operator=<=  OutDataTypeStr=boolean  RndMeth=Simplest
  Timer1 : Subsystem
  Out1 : Outport
  wires:
  Timer1/2(counter_status) -> "Latch "/1(Input)
  Timer1/1(counter out) -> Relational Operator16/1
  LatchResetCounterVal/1 -> Relational Operator16/2
  incrcondition/1 -> Timer1/1(incrcondition)
  incrvalue/1 -> Timer1/2(incrvalue)
  Relational Operator16/1 -> "Latch "/2(Latch Reset)
  "Latch "/1(Output) -> Out1/1
  maxlimit/1 -> Timer1/5(maxlimit)
  decrcondition/1 -> Timer1/3(decrcondition)
  reset/1 -> Timer1/6(reset)
  decvalue/1 -> Timer1/4(decvalue)

== system ADIA/ADAS_Diagnostics/Diagnostics_Processing/Rationality_Diagnostics/DTC_EMS_14A_OorACCStatus/Counter&Latch ==
  incrcondition : Inport
  incrvalue : Inport  Port=2
  decrcondition : Inport  Port=3
  decvalue : Inport  Port=4
  maxlimit : Inport  Port=5
  reset : Inport  Port=6
  LatchResetCounterVal : Inport  Port=7
  "Latch " : Subsystem
  Relational Operator16 : RelationalOperator  Operator=<=  OutDataTypeStr=boolean  RndMeth=Simplest
  Timer1 : Subsystem
  Out1 : Outport
  wires:
  Timer1/2(counter_status) -> "Latch "/1(Input)
  Timer1/1(counter out) -> Relational Operator16/1
  LatchResetCounterVal/1 -> Relational Operator16/2
  incrcondition/1 -> Timer1/1(incrcondition)
  incrvalue/1 -> Timer1/2(incrvalue)
  Relational Operator16/1 -> "Latch "/2(Latch Reset)
  "Latch "/1(Output) -> Out1/1
  maxlimit/1 -> Timer1/5(maxlimit)
  decrcondition/1 -> Timer1/3(decrcondition)
  reset/1 -> Timer1/6(reset)
  decvalue/1 -> Timer1/4(decvalue)

== system ADIA/ADAS_Diagnostics/Diagnostics_Processing/Rationality_Diagnostics/DTC_WheelSpdFaultSignal/Counter&Latch ==
  incrcondition : Inport
  incrvalue : Inport  Port=2
  decrcondition : Inport  Port=3
  decvalue : Inport  Port=4
  maxlimit : Inport  Port=5
  reset : Inport  Port=6
  LatchResetCounterVal : Inport  Port=7
  "Latch " : Subsystem
  Relational Operator16 : RelationalOperator  Operator=<=  OutDataTypeStr=boolean  RndMeth=Simplest
  Timer1 : Subsystem
  Out1 : Outport
  wires:
  Timer1/2(counter_status) -> "Latch "/1(Input)
  Timer1/1(counter out) -> Relational Operator16/1
  LatchResetCounterVal/1 -> Relational Operator16/2
  incrcondition/1 -> Timer1/1(incrcondition)
  incrvalue/1 -> Timer1/2(incrvalue)
  Relational Operator16/1 -> "Latch "/2(Latch Reset)
  "Latch "/1(Output) -> Out1/1
  maxlimit/1 -> Timer1/5(maxlimit)
  decrcondition/1 -> Timer1/3(decrcondition)
  reset/1 -> Timer1/6(reset)
  decvalue/1 -> Timer1/4(decvalue)

== system ADIA/ADAS_Diagnostics/Diagnostics_Processing/Rationality_Diagnostics/EMS10_88_InvAccPedPosRaw/Counter&Latch ==
  incrcondition : Inport
  incrvalue : Inport  Port=2
  decrcondition : Inport  Port=3
  decvalue : Inport  Port=4
  maxlimit : Inport  Port=5
  reset : Inport  Port=6
  LatchResetCounterVal : Inport  Port=7
  "Latch " : Subsystem
  Relational Operator16 : RelationalOperator  Operator=<=  OutDataTypeStr=boolean  RndMeth=Simplest
  Timer1 : Subsystem
  Out1 : Outport
  wires:
  Timer1/2(counter_status) -> "Latch "/1(Input)
  Timer1/1(counter out) -> Relational Operator16/1
  LatchResetCounterVal/1 -> Relational Operator16/2
  incrcondition/1 -> Timer1/1(incrcondition)
  incrvalue/1 -> Timer1/2(incrvalue)
  Relational Operator16/1 -> "Latch "/2(Latch Reset)
  "Latch "/1(Output) -> Out1/1
  maxlimit/1 -> Timer1/5(maxlimit)
  decrcondition/1 -> Timer1/3(decrcondition)
  reset/1 -> Timer1/6(reset)
  decvalue/1 -> Timer1/4(decvalue)

== system ADIA/ADAS_Diagnostics/Diagnostics_Processing/Rationality_Diagnostics/EMS5_E0_InvOorBrkPedal/Counter&Latch ==
  incrcondition : Inport
  incrvalue : Inport  Port=2
  decrcondition : Inport  Port=3
  decvalue : Inport  Port=4
  maxlimit : Inport  Port=5
  reset : Inport  Port=6
  LatchResetCounterVal : Inport  Port=7
  "Latch " : Subsystem
  Relational Operator16 : RelationalOperator  Operator=<=  OutDataTypeStr=boolean  RndMeth=Simplest
  Timer1 : Subsystem
  Out1 : Outport
  wires:
  Timer1/2(counter_status) -> "Latch "/1(Input)
  Timer1/1(counter out) -> Relational Operator16/1
  LatchResetCounterVal/1 -> Relational Operator16/2
  incrcondition/1 -> Timer1/1(incrcondition)
  incrvalue/1 -> Timer1/2(incrvalue)
  Relational Operator16/1 -> "Latch "/2(Latch Reset)
  "Latch "/1(Output) -> Out1/1
  maxlimit/1 -> Timer1/5(maxlimit)
  decrcondition/1 -> Timer1/3(decrcondition)
  reset/1 -> Timer1/6(reset)
  decvalue/1 -> Timer1/4(decvalue)

== system ADIA/ADAS_Diagnostics/Diagnostics_Processing/Rationality_Diagnostics/EMS5_E0_OorEngineStas/Counter&Latch ==
  incrcondition : Inport
  incrvalue : Inport  Port=2
  decrcondition : Inport  Port=3
  decvalue : Inport  Port=4
  maxlimit : Inport  Port=5
  reset : Inport  Port=6
  LatchResetCounterVal : Inport  Port=7
  "Latch " : Subsystem
  Relational Operator16 : RelationalOperator  Operator=<=  OutDataTypeStr=boolean  RndMeth=Simplest
  Timer1 : Subsystem
  Out1 : Outport
  wires:
  Timer1/2(counter_status) -> "Latch "/1(Input)
  Timer1/1(counter out) -> Relational Operator16/1
  LatchResetCounterVal/1 -> Relational Operator16/2
  incrcondition/1 -> Timer1/1(incrcondition)
  incrvalue/1 -> Timer1/2(incrvalue)
  Relational Operator16/1 -> "Latch "/2(Latch Reset)
  "Latch "/1(Output) -> Out1/1
  maxlimit/1 -> Timer1/5(maxlimit)
  decrcondition/1 -> Timer1/3(decrcondition)
  reset/1 -> Timer1/6(reset)
  decvalue/1 -> Timer1/4(decvalue)

== system ADIA/ADAS_Diagnostics/Diagnostics_Processing/Rationality_Diagnostics/EMS_14B_InvOorRealWhlTrq/Counter&Latch ==
  incrcondition : Inport
  incrvalue : Inport  Port=2
  decrcondition : Inport  Port=3
  decvalue : Inport  Port=4
  maxlimit : Inport  Port=5
  reset : Inport  Port=6
  LatchResetCounterVal : Inport  Port=7
  "Latch " : Subsystem
  Relational Operator16 : RelationalOperator  Operator=<=  OutDataTypeStr=boolean  RndMeth=Simplest
  Timer1 : Subsystem
  Out1 : Outport
  wires:
  Timer1/2(counter_status) -> "Latch "/1(Input)
  Timer1/1(counter out) -> Relational Operator16/1
  LatchResetCounterVal/1 -> Relational Operator16/2
  incrcondition/1 -> Timer1/1(incrcondition)
  incrvalue/1 -> Timer1/2(incrvalue)
  Relational Operator16/1 -> "Latch "/2(Latch Reset)
  "Latch "/1(Output) -> Out1/1
  maxlimit/1 -> Timer1/5(maxlimit)
  decrcondition/1 -> Timer1/3(decrcondition)
  reset/1 -> Timer1/6(reset)
  decvalue/1 -> Timer1/4(decvalue)

== system ADIA/ADAS_Diagnostics/Diagnostics_Processing/Rationality_Diagnostics/EMS_17E_InvOorMaxNoCtrlTrq/Counter&Latch ==
  incrcondition : Inport
  incrvalue : Inport  Port=2
  decrcondition : Inport  Port=3
  decvalue : Inport  Port=4
  maxlimit : Inport  Port=5
  reset : Inport  Port=6
  LatchResetCounterVal : Inport  Port=7
  "Latch " : Subsystem
  Relational Operator16 : RelationalOperator  Operator=<=  OutDataTypeStr=boolean  RndMeth=Simplest
  Timer1 : Subsystem
  Out1 : Outport
  wires:
  Timer1/2(counter_status) -> "Latch "/1(Input)
  Timer1/1(counter out) -> Relational Operator16/1
  LatchResetCounterVal/1 -> Relational Operator16/2
  incrcondition/1 -> Timer1/1(incrcondition)
  incrvalue/1 -> Timer1/2(incrvalue)
  Relational Operator16/1 -> "Latch "/2(Latch Reset)
  "Latch "/1(Output) -> Out1/1
  maxlimit/1 -> Timer1/5(maxlimit)
  decrcondition/1 -> Timer1/3(decrcondition)
  reset/1 -> Timer1/6(reset)
  decvalue/1 -> Timer1/4(decvalue)

== system ADIA/ADAS_Diagnostics/Diagnostics_Processing/Rationality_Diagnostics/EMS_17E_InvOorMaxTrqWhl/Counter&Latch ==
  incrcondition : Inport
  incrvalue : Inport  Port=2
  decrcondition : Inport  Port=3
  decvalue : Inport  Port=4
  maxlimit : Inport  Port=5
  reset : Inport  Port=6
  LatchResetCounterVal : Inport  Port=7
  "Latch " : Subsystem
  Relational Operator16 : RelationalOperator  Operator=<=  OutDataTypeStr=boolean  RndMeth=Simplest
  Timer1 : Subsystem
  Out1 : Outport
  wires:
  Timer1/2(counter_status) -> "Latch "/1(Input)
  Timer1/1(counter out) -> Relational Operator16/1
  LatchResetCounterVal/1 -> Relational Operator16/2
  incrcondition/1 -> Timer1/1(incrcondition)
  incrvalue/1 -> Timer1/2(incrvalue)
  Relational Operator16/1 -> "Latch "/2(Latch Reset)
  "Latch "/1(Output) -> Out1/1
  maxlimit/1 -> Timer1/5(maxlimit)
  decrcondition/1 -> Timer1/3(decrcondition)
  reset/1 -> Timer1/6(reset)
  decvalue/1 -> Timer1/4(decvalue)

== system ADIA/ADAS_Diagnostics/Diagnostics_Processing/Rationality_Diagnostics/EMS_17E_InvOorMinNoCtrlTrq/Counter&Latch ==
  incrcondition : Inport
  incrvalue : Inport  Port=2
  decrcondition : Inport  Port=3
  decvalue : Inport  Port=4
  maxlimit : Inport  Port=5
  reset : Inport  Port=6
  LatchResetCounterVal : Inport  Port=7
  "Latch " : Subsystem
  Relational Operator16 : RelationalOperator  Operator=<=  OutDataTypeStr=boolean  RndMeth=Simplest
  Timer1 : Subsystem
  Out1 : Outport
  wires:
  Timer1/2(counter_status) -> "Latch "/1(Input)
  Timer1/1(counter out) -> Relational Operator16/1
  LatchResetCounterVal/1 -> Relational Operator16/2
  incrcondition/1 -> Timer1/1(incrcondition)
  incrvalue/1 -> Timer1/2(incrvalue)
  Relational Operator16/1 -> "Latch "/2(Latch Reset)
  "Latch "/1(Output) -> Out1/1
  maxlimit/1 -> Timer1/5(maxlimit)
  decrcondition/1 -> Timer1/3(decrcondition)
  reset/1 -> Timer1/6(reset)
  decvalue/1 -> Timer1/4(decvalue)

== system ADIA/ADAS_Diagnostics/Diagnostics_Processing/Rationality_Diagnostics/EMS_17E_InvOorMinTrqWhl/Counter&Latch ==
  incrcondition : Inport
  incrvalue : Inport  Port=2
  decrcondition : Inport  Port=3
  decvalue : Inport  Port=4
  maxlimit : Inport  Port=5
  reset : Inport  Port=6
  LatchResetCounterVal : Inport  Port=7
  "Latch " : Subsystem
  Relational Operator16 : RelationalOperator  Operator=<=  OutDataTypeStr=boolean  RndMeth=Simplest
  Timer1 : Subsystem
  Out1 : Outport
  wires:
  Timer1/2(counter_status) -> "Latch "/1(Input)
  Timer1/1(counter out) -> Relational Operator16/1
  LatchResetCounterVal/1 -> Relational Operator16/2
  incrcondition/1 -> Timer1/1(incrcondition)
  incrvalue/1 -> Timer1/2(incrvalue)
  Relational Operator16/1 -> "Latch "/2(Latch Reset)
  "Latch "/1(Output) -> Out1/1
  maxlimit/1 -> Timer1/5(maxlimit)
  decrcondition/1 -> Timer1/3(decrcondition)
  reset/1 -> Timer1/6(reset)
  decvalue/1 -> Timer1/4(decvalue)

== system ADIA/ADAS_Diagnostics/Diagnostics_Processing/Rationality_Diagnostics/EPS2_17A_InvOorSteAngle/Counter&Latch ==
  incrcondition : Inport
  incrvalue : Inport  Port=2
  decrcondition : Inport  Port=3
  decvalue : Inport  Port=4
  maxlimit : Inport  Port=5
  reset : Inport  Port=6
  LatchResetCounterVal : Inport  Port=7
  "Latch " : Subsystem
  Relational Operator16 : RelationalOperator  Operator=<=  OutDataTypeStr=boolean  RndMeth=Simplest
  Timer1 : Subsystem
  Out1 : Outport
  wires:
  Timer1/2(counter_status) -> "Latch "/1(Input)
  Timer1/1(counter out) -> Relational Operator16/1
  LatchResetCounterVal/1 -> Relational Operator16/2
  incrcondition/1 -> Timer1/1(incrcondition)
  incrvalue/1 -> Timer1/2(incrvalue)
  Relational Operator16/1 -> "Latch "/2(Latch Reset)
  "Latch "/1(Output) -> Out1/1
  maxlimit/1 -> Timer1/5(maxlimit)
  decrcondition/1 -> Timer1/3(decrcondition)
  reset/1 -> Timer1/6(reset)
  decvalue/1 -> Timer1/4(decvalue)

== system ADIA/ADAS_Diagnostics/Diagnostics_Processing/Rationality_Diagnostics/EPS2_17A_InvStTorq/Counter&Latch ==
  incrcondition : Inport
  incrvalue : Inport  Port=2
  decrcondition : Inport  Port=3
  decvalue : Inport  Port=4
  maxlimit : Inport  Port=5
  reset : Inport  Port=6
  LatchResetCounterVal : Inport  Port=7
  "Latch " : Subsystem
  Relational Operator16 : RelationalOperator  Operator=<=  OutDataTypeStr=boolean  RndMeth=Simplest
  Timer1 : Subsystem
  Out1 : Outport
  wires:
  Timer1/2(counter_status) -> "Latch "/1(Input)
  Timer1/1(counter out) -> Relational Operator16/1
  LatchResetCounterVal/1 -> Relational Operator16/2
  incrcondition/1 -> Timer1/1(incrcondition)
  incrvalue/1 -> Timer1/2(incrvalue)
  Relational Operator16/1 -> "Latch "/2(Latch Reset)
  "Latch "/1(Output) -> Out1/1
  maxlimit/1 -> Timer1/5(maxlimit)
  decrcondition/1 -> Timer1/3(decrcondition)
  reset/1 -> Timer1/6(reset)
  decvalue/1 -> Timer1/4(decvalue)

== system ADIA/ADAS_Diagnostics/Diagnostics_Processing/Rationality_Diagnostics/EPS3_31C_InvOorLKAState/Counter&Latch ==
  incrcondition : Inport
  incrvalue : Inport  Port=2
  decrcondition : Inport  Port=3
  decvalue : Inport  Port=4
  maxlimit : Inport  Port=5
  reset : Inport  Port=6
  LatchResetCounterVal : Inport  Port=7
  "Latch " : Subsystem
  Relational Operator16 : RelationalOperator  Operator=<=  OutDataTypeStr=boolean  RndMeth=Simplest
  Timer1 : Subsystem
  Out1 : Outport
  wires:
  Timer1/2(counter_status) -> "Latch "/1(Input)
  Timer1/1(counter out) -> Relational Operator16/1
  LatchResetCounterVal/1 -> Relational Operator16/2
  incrcondition/1 -> Timer1/1(incrcondition)
  incrvalue/1 -> Timer1/2(incrvalue)
  Relational Operator16/1 -> "Latch "/2(Latch Reset)
  "Latch "/1(Output) -> Out1/1
  maxlimit/1 -> Timer1/5(maxlimit)
  decrcondition/1 -> Timer1/3(decrcondition)
  reset/1 -> Timer1/6(reset)
  decvalue/1 -> Timer1/4(decvalue)

== system ADIA/ADAS_Diagnostics/Diagnostics_Processing/Rationality_Diagnostics/ESC2_A0_InvOorVehSpeed/Counter&Latch ==
  incrcondition : Inport
  incrvalue : Inport  Port=2
  decrcondition : Inport  Port=3
  decvalue : Inport  Port=4
  maxlimit : Inport  Port=5
  reset : Inport  Port=6
  LatchResetCounterVal : Inport  Port=7
  "Latch " : Subsystem
  Relational Operator16 : RelationalOperator  Operator=<=  OutDataTypeStr=boolean  RndMeth=Simplest
  Timer1 : Subsystem
  Out1 : Outport
  wires:
  Timer1/2(counter_status) -> "Latch "/1(Input)
  Timer1/1(counter out) -> Relational Operator16/1
  LatchResetCounterVal/1 -> Relational Operator16/2
  incrcondition/1 -> Timer1/1(incrcondition)
  incrvalue/1 -> Timer1/2(incrvalue)
  Relational Operator16/1 -> "Latch "/2(Latch Reset)
  "Latch "/1(Output) -> Out1/1
  maxlimit/1 -> Timer1/5(maxlimit)
  decrcondition/1 -> Timer1/3(decrcondition)
  reset/1 -> Timer1/6(reset)
  decvalue/1 -> Timer1/4(decvalue)

== system ADIA/ADAS_Diagnostics/Diagnostics_Processing/Rationality_Diagnostics/ESC3_121_InvOorTCSActive/Counter&Latch ==
  incrcondition : Inport
  incrvalue : Inport  Port=2
  decrcondition : Inport  Port=3
  decvalue : Inport  Port=4
  maxlimit : Inport  Port=5
  reset : Inport  Port=6
  LatchResetCounterVal : Inport  Port=7
  "Latch " : Subsystem
  Relational Operator16 : RelationalOperator  Operator=<=  OutDataTypeStr=boolean  RndMeth=Simplest
  Timer1 : Subsystem
  Out1 : Outport
  wires:
  Timer1/2(counter_status) -> "Latch "/1(Input)
  Timer1/1(counter out) -> Relational Operator16/1
  LatchResetCounterVal/1 -> Relational Operator16/2
  incrcondition/1 -> Timer1/1(incrcondition)
  incrvalue/1 -> Timer1/2(incrvalue)
  Relational Operator16/1 -> "Latch "/2(Latch Reset)
  "Latch "/1(Output) -> Out1/1
  maxlimit/1 -> Timer1/5(maxlimit)
  decrcondition/1 -> Timer1/3(decrcondition)
  reset/1 -> Timer1/6(reset)
  decvalue/1 -> Timer1/4(decvalue)
